simulink model "sldemo_drivecycle_org"  (Simulink 10.0)
settings: Solver=ode45  StartTime=0.0  StopTime=1e5  MaxStep=1  RelTol=1e-3  EnableMultiTasking=on
libraries: drivecyclelib x1
settings Model: Creator=e102261  LastModifiedBy=bhisma
settings DataIOCC: LimitDataPoints=on  SaveOutput=off  SignalLogging=off  DSMLogging=off  SaveTime=off
settings OptimizationCC: ExpressionDepthLimit=2147483647
settings DebuggingCC: SolverPrmCheckMsg=warning  MultiTaskDSMMsg=warning  MultiTaskCondExecSysMsg=none  FcnCallInpInsideContextMsg=warning  StateNameClashWarn=warning  SFExecutionAtInitializationDiag=warning
settings GRTTargetCC: GeneratePreprocessorConditionals=Disable all  CombineOutputUpdateFcns=on  GRTInterface=off
settings ConfigComp: CovExternalEMLEnable=off

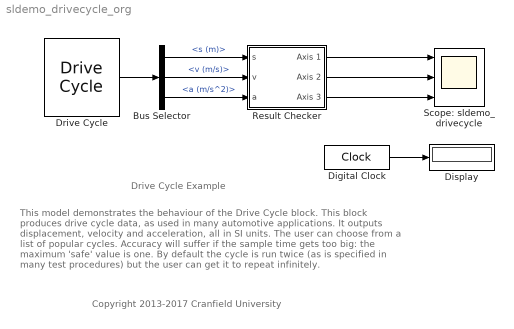
== system sldemo_drivecycle_org ==
  note: This model demonstrates the behaviour of the Drive Cycle block.  This block
      | produces drive cycle data, as used in many automotive applications.  It
      | outputs displacement, velocity and acceleration, all in SI units.  The user can
      | choose from a list of popular cycles. Accuracy will suffer if the sample time gets
      | too big: the maximum 'safe' value is one.  By default the cycle is run twice (as
      | is specified in many test procedures) but the user can get it to repeat infinitely.
  note: Drive Cycle Example
  note: Copyright 2013-2017 Cranfield University
  Bus Selector : BusSelector  OutputSignals=s (m),v (m/s),a (m/s^2)
  Digital Clock : DigitalClock
  Display : Display
  Drive Cycle : drivecyclelib/Drive Cycle  CycleName=WLTP class 3  CycleRepeatsForever=off
  Result Checker : Subsystem
  Scope: sldemo_drivecycle : Scope  NumInputPorts=3
  wires:
  Result Checker/1(Axis 1) -> Scope: sldemo_drivecycle/1
  Result Checker/2(Axis 2) -> Scope: sldemo_drivecycle/2
  Result Checker/3(Axis 3) -> Scope: sldemo_drivecycle/3
  Drive Cycle/1 -> Bus Selector/1
  Bus Selector/1 -> Result Checker/1(s)  "<s (m)>"
  Bus Selector/2 -> Result Checker/2(v)  "<v (m/s)>"
  Bus Selector/3 -> Result Checker/3(a)  "<a (m/s^2)>"
  Digital Clock/1 -> Display/1

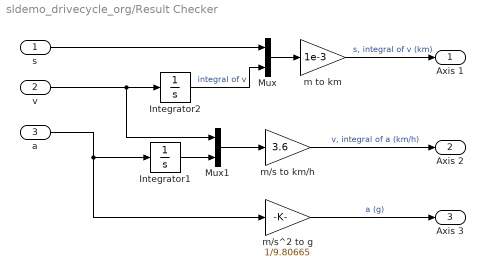
== system sldemo_drivecycle_org/Result Checker ==
  s : Inport
  v : Inport  Port=2
  a : Inport  Port=3
  Integrator1 : Integrator
  Integrator2 : Integrator
  Mux : Mux  Inputs=2
  Mux1 : Mux  Inputs=2
  m to km : Gain  Gain=1e-3
  m/s to km/h : Gain  Gain=3.6
  m/s^2 to g : Gain  Gain=1/9.80665
  Axis 1 : Outport
  Axis 2 : Outport  Port=2
  Axis 3 : Outport  Port=3
  wires:
  Mux/1 -> m to km/1
  Integrator1/1 -> Mux1/2
  Integrator2/1 -> Mux/2  "integral of v"
  Mux1/1 -> m/s to km/h/1
  v/1 -> Integrator2/1, Mux1/1
  a/1 -> m/s^2 to g/1, Integrator1/1
  s/1 -> Mux/1
  m to km/1 -> Axis 1/1  "s, integral of v (km)"
  m/s to km/h/1 -> Axis 2/1  "v, integral of a (km/h)"
  m/s^2 to g/1 -> Axis 3/1  "a (g)"
